simulink model "KalmanPendulumSim"  (R2018b)
settings: Solver=VariableStepAuto  StartTime=0.0  StopTime=10  FixedStep=dt  RelTol=1e-3
model workspace (MAT data in the model file):
  ControlTs = 0.01
  FNorm = 3
  L = 1
  Omega0 = 0
  OmegaNorm = 3
  Q = [0  0; 0  0.0174532925199]
  R = 1.11111111111e-07
  Theta0 = 1.0471975512
  dx = 0.001
  g = 9.81
  l = 1
  m = 1
undefined symbols (not defined in the file): DiscIntNeverNeededParam, Discrete, Time
libraries: simulink x1, sharedTrackingLibrary x1, ctrlSharedLib x1, dspsrcs4 x1, aerolibanimutils x1
settings Model: Creator=alons  LastModifiedBy=alons

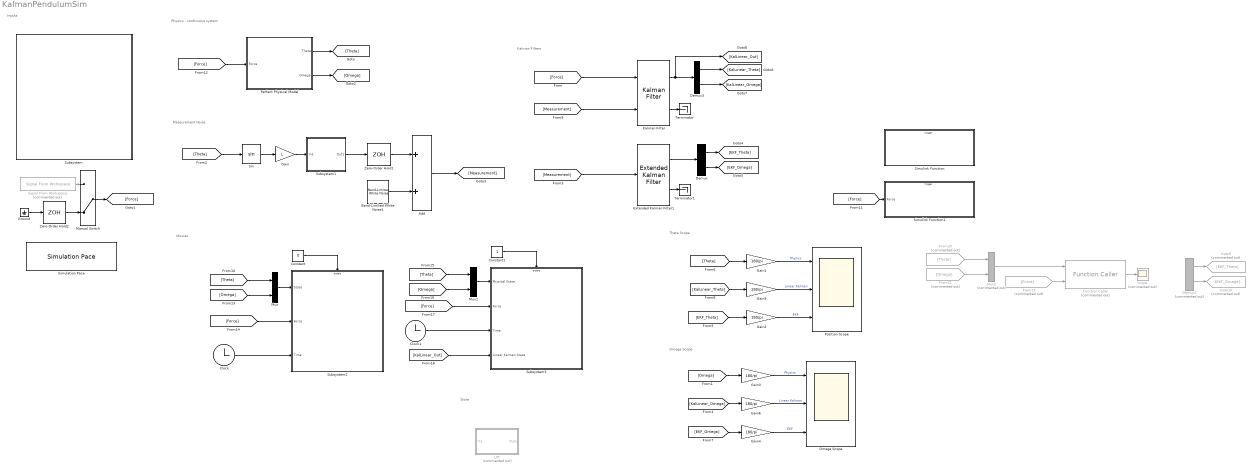
== system KalmanPendulumSim ==
  note: Store
  note: Movies
  note: Theta Scope
  note: Measurement Noise
  note: Physics - continuous system
  note: Kalman Filters
  note: Omega Scope
  note: Inputs
  Add : Sum
  Band-Limited White Noise1 : simulink/Sources/Band-Limited White Noise  Cov=R  Ts=ControlTs  seed=[23341]
  Clock : Clock
  Clock1 : Clock
  Constant : Constant  Value=0  SampleTime=0
      settings: OpenFcn=|
      | if get_param(gcbh,'value')-48
      |    set_param(gcbh,'value','0','backgroundcolor','red');
      | else
      |    set_param(gcbh,'value','1','backgroundcolor','green');
      | end
  Constant1 : Constant  SampleTime=0
      settings: OpenFcn=|
      | if get_param(gcbh,'value')-48
      |    set_param(gcbh,'value','0','backgroundcolor','red');
      | else
      |    set_param(gcbh,'value','1','backgroundcolor','green');
      | end
  Demux : Demux  Outputs=2
  Demux2 : Demux  Commented=on  Outputs=2
  Demux3 : Demux  Outputs=2
  Extended Kalman Filter1 : sharedTrackingLibrary/Extended Kalman Filter  StateTransitionFcn=StateTransition  HasStateTransitionJacobianFcn=off  HasAdditiveProcessNoise=Additive  ProcessNoise=Q  HasTimeVaryingProcessNoise=off  HasStateTransitionFcnExtraArgument=0  InitialState=[Theta0;Omega0]  InitialStateCovariance=zeros(2,2)  MeasurementFcn1=Measurement2Theta  HasMeasurementJacobianFcn1=off  HasMeasurementEnablePort1=off  HasAdditiveMeasurementNoise1=Additive  MeasurementNoise1=R  HasTimeVaryingMeasurementNoise1=off  HasMeasurementFcnExtraArgument1=0  MeasurementFcn2=myMeasurementFcn  HasMeasurementJacobianFcn2=off  HasMeasurementEnablePort2=off  HasAdditiveMeasurementNoise2=Additive  MeasurementNoise2=1  HasTimeVaryingMeasurementNoise2=off  HasMeasurementFcnExtraArgument2=0  MeasurementFcn3=myMeasurementFcn  HasMeasurementJacobianFcn3=off  HasMeasurementEnablePort3=off  HasAdditiveMeasurementNoise3=Additive  MeasurementNoise3=1  HasTimeVaryingMeasurementNoise3=off  HasMeasurementFcnExtraArgument3=0  MeasurementFcn4=myMeasurementFcn  HasMeasurementJacobianFcn4=off  HasMeasurementEnablePort4=off  HasAdditiveMeasurementNoise4=Additive  MeasurementNoise4=1  HasTimeVaryingMeasurementNoise4=off  HasMeasurementFcnExtraArgument4=0  MeasurementFcn5=myMeasurementFcn  HasMeasurementJacobianFcn5=off  HasMeasurementEnablePort5=off  HasAdditiveMeasurementNoise5=Additive  MeasurementNoise5=1  HasTimeVaryingMeasurementNoise5=off  HasMeasurementFcnExtraArgument5=0  EnableMultirate=off  StateTransitionFcnSampleTime=1  MeasurementFcn1SampleTime=1  MeasurementFcn2SampleTime=1  MeasurementFcn3SampleTime=1  MeasurementFcn4SampleTime=1  MeasurementFcn5SampleTime=1  UseCurrentEstimator=on  OutputStateCovariance=on  DataType=double  SampleTime=ControlTs  NumberOfMeasurements=1
      settings: SourceProductName=Control System Toolbox  SourceProductBaseCode=CT
  From19 : From  Commented=on  GotoTag=Force
  From20 : From  Commented=on  GotoTag=Theta
  From21 : From  Commented=on  GotoTag=Omega
  Function Caller : FunctionCaller  Commented=on  FunctionPrototype=x_kp1 = StateTransition(x_k,Force)
  Gain : Gain  Gain=L
  Gain{1..6} (6 alike) : Gain  Gain=180/pi
  Goto10 : Goto  Commented=on  GotoTag=EKF_Omega
  Goto9 : Goto  Commented=on  GotoTag=EKF_Theta
  Ground : Ground
  Kalman Filter : ctrlSharedLib/Kalman Filter  TimeDomain=Discrete-Time  UseCurrentEstimator=on  ModelSource=Individual A, B, C, D matrices  ModelSourceVariable=ss(0.95,1,1,0,1)  A=[0,1;-sqrt(g/L),0]  B=zeros(2,1)  C=[L,0]  D=0  NumberOfStates=1  NumberOfInputs=1  NumberOfOutputs=1  InitialEstimateSource=Dialog  X0=[Theta0,Omega0]  P0=10  UseK=off  UseGH=off  NumberOfProcessNoiseInputs=1  G=1  TimeInvariantG=on  H=0  TimeInvariantH=on  Q=Q  TimeInvariantQ=on  R=R  TimeInvariantR=on  N=0  TimeInvariantN=on  AddInputPort=on  AddEnablePort=off  OutputEstimatedY=off  OutputP=on  Ts=-1
      settings: SourceProductBaseCode=CT
  LPF : Subsystem  Commented=on  mask{Freq=1000}
      mask prompts: Freq "LPF Freq [Hz]"
      mask Display: fprintf('LPF %g[Hz]',Freq);
  Manual Switch : ManualSwitch  CurrentSetting=0
  Mux : Mux  Inputs=2
  Mux1 : Mux  Inputs=2
  Mux2 : Mux  Commented=on  Inputs=2
  Omega Scope : Scope  NumInputPorts=3
  Perfect Physical Model : Subsystem
  Position Scope : Scope  NumInputPorts=3
  Scope : Scope  Commented=on
  Signal From Workspace : dspsrcs4/Signal From Workspace  Commented=on  X=F  Ts=ControlTs  nsamps=1  OutputAfterFinalValue=Setting to zero  ignoreOrWarnInputAndFrameLengths=off  OutputFrames=off
  Simulation Pace : aerolibanimutils/Simulation Pace  SimulationPace=1  SleepMode=Auto  OutputPaceError=off  SampleTime=ControlTs
  Simulink Function : Subsystem  TreatAsAtomicUnit=on
  Simulink Function1 : Subsystem  TreatAsAtomicUnit=on
  Sin : Trigonometry
  Subsystem : Subsystem  InitFcn=|  mask{ControlTs=0.01, L=1, m=1, dx=1*10^-3, g=9.81, Theta0=60*pi/180, Omega0=0*pi/180, Q=diag([0,1])*pi/180, R=((1*10^-3)/3)^2, FNorm=3, OmegaNorm=3}
      | mdlWks=get_param(bdroot,'ModelWorkspace')
      | par = get_param(gcb,'DialogParameters');
      | fnames = fieldnames(par);
      | for ipar=1:length(fnames)
      |    num=str2num(get_param(gcb,fnames{ipar}));
      |    mdlWks.assignin(fnames{ipar},num);
      | end
      | 
      | clear par fnames ipar num mdlWks;
      mask prompts: ControlTs "Control Time Sample [s]"; L "String Length [m]"; m "Bolb Mass [kg]"; dx "dx - Encoder Resolution [m]"; g "g - gravity acceleration [m/s^2]"; Theta0 "Initial Theta [rad]"; Omega0 "Initial Omega [rad/s]"; Q "Q - Model Noise Covaraince [rad,rad/s]"; R "R - Measuremnt Noise Covariance"; FNorm "FNorm - for drawing [N]"; OmegaNorm "OmegaNorm - for drawing [rad/s]"
      mask Display:
      | str=[
      |     'Model Workspace Parameters \n\n\n',...
      |     'ControlTs = %g[s]\n\n',...
      |     'm = %g[kg]\n\n',...
      |     'L = %g[m]\n\n',...
      |     'dx = %g[m]\n\n\n',...
      |     'g = %g[m/s^2]\n\n',...
      |     'Theta0 = %g[rad]\n\n',...
      |     'Omega0 = %g[rad/s]\n\n',...
      |     'Q(1,1) = %g[rad]\n\n',...
      |     'Q(2,2) = %g[rad/s]\n\n',...
      |     'R = %g[m]\n\n\n',...
      |     'For Drawing\n\n',...
      |     'FNorm = %g[N]\n\n',...
      |     'OmegaNorm = %g[rad/s]',...
      |     ];
      | fprintf(str,ControlTs,m,L,dx,g,Theta0,...
      |     Omega0,Q(1,1),Q(2,2),R,FNorm,OmegaNorm);
  Subsystem1 : Subsystem
      mask Display: disp('Physics 2 Resolution')
  Subsystem2 : Subsystem
      settings: OpenFcn=|
      | UserData = get_param([gcb,'/AnimationSfcn'],'UserData');
      | Fig = UserData.Figure;
      | if ishghandle(Fig,'figure');
      |    %bring to the front:
      |    figure(Fig);
      | end
      mask Display:
      | t=linspace(0,2*pi,20);
      | plot(cos(t),sin(t));
      | 
      | x=[-0.4,-0.4,0.6,-0.4];
      | y=[-0.5,0.5,0,-0.5];
      | plot(x,y)
      | 
      | disp('Physical System')
  Subsystem3 : Subsystem
      settings: OpenFcn=|
      | UserData = get_param([gcb,'/AnimationSfcn'],'UserData');
      | Fig = UserData.Figure;
      | if ishghandle(Fig,'figure');
      |    %bring to the front:
      |    figure(Fig);
      | end
      mask Display:
      | t=linspace(0,2*pi,20);
      | plot(cos(t),sin(t));
      | 
      | x=[-0.4,-0.4,0.6,-0.4];
      | y=[-0.5,0.5,0,-0.5];
      | plot(x,y)
      | 
      | disp('Linear Kalman System')
  Terminator : Terminator
  Terminator1 : Terminator
  Zero-Order Hold1 : ZeroOrderHold  SampleTime=ControlTs
  Zero-Order Hold2 : ZeroOrderHold  SampleTime=ControlTs
  wires:
  [Theta] -> Sin/1
  Sin/1 -> Gain/1
  Extended Kalman Filter1/1 -> Demux/1
  Band-Limited White Noise1/1 -> Add/2
  Demux/1 -> [EKF_Theta]
  Demux/2 -> [EKF_Omega]
  [EKF_Theta] -> Gain2/1
  [Theta] -> Gain1/1
  Gain1/1 -> Position Scope/1  "Physics"
  [Omega] -> Gain3/1
  [EKF_Omega] -> Gain4/1
  Gain3/1 -> Omega Scope/1  "Physics"
  Demux3/1 -> [KalLinear_Theta]
  Demux3/2 -> [KalLinear_Omega]
  Kalman Filter/1 -> Demux3/1, [KalLinear_Out]
  [KalLinear_Theta] -> Gain5/1
  Gain2/1 -> Position Scope/3  "EKF"
  Gain5/1 -> Position Scope/2  "Linear Kalman"
  Gain4/1 -> Omega Scope/3  "EKF"
  [KalLinear_Omega] -> Gain6/1
  Gain6/1 -> Omega Scope/2  "Linear Kalman"
  [Measurement] -> Kalman Filter/2
  [Measurement] -> Extended Kalman Filter1/1
  Signal From Workspace/1 -> Manual Switch/1
  Ground/1 -> Zero-Order Hold2/1
  Manual Switch/1 -> [Force]
  [Force] -> Perfect Physical Model/1(Force)
  Perfect Physical Model/1(Theta) -> [Theta]
  Perfect Physical Model/2(Omega) -> [Omega]
  [Force] -> Kalman Filter/1
  Gain/1 -> Subsystem1/1(In1)
  Add/1 -> [Measurement]
  Subsystem1/1(Out1) -> Zero-Order Hold1/1
  Zero-Order Hold1/1 -> Add/1
  [Theta] -> Mux/1
  Clock/1 -> Subsystem2/3(Time)
  [Force] -> Subsystem2/2(Force)
  Mux/1 -> Subsystem2/1(State)
  [Omega] -> Mux/2
  Constant/1 -> Subsystem2/Enable
  Zero-Order Hold2/1 -> Manual Switch/2
  Constant1/1 -> Subsystem3/Enable
  [Omega] -> Mux1/2
  Clock1/1 -> Subsystem3/3(Time)
  [Theta] -> Mux1/1
  [Force] -> Subsystem3/2(Force)
  Mux1/1 -> Subsystem3/1(Physical State)
  [KalLinear_Out] -> Subsystem3/4(Linear Kalman State)
  From19/1 -> Function Caller/2
  From21/1 -> Mux2/2
  From20/1 -> Mux2/1
  Demux2/2 -> Goto10/1
  Demux2/1 -> Goto9/1
  Function Caller/1 -> Scope/1
  Mux2/1 -> Function Caller/1
  [Force] -> Simulink Function1/1(Force)
  Kalman Filter/2 -> Terminator/1
  Extended Kalman Filter1/2 -> Terminator1/1

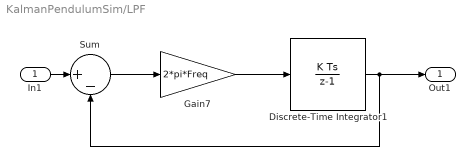
== system KalmanPendulumSim/LPF ==
  In1 : Inport
  Discrete-Time Integrator1 : DiscreteIntegrator  SampleTime=-1  ICPrevOutput=DiscIntNeverNeededParam  ICPrevScaledInput=DiscIntNeverNeededParam
  Gain7 : Gain  Gain=2*pi*Freq
  Sum : Sum  Inputs=|+-
  Out1 : Outport
  wires:
  Discrete-Time Integrator1/1 -> Out1/1, Sum/2
  Sum/1 -> Gain7/1
  Gain7/1 -> Discrete-Time Integrator1/1
  In1/1 -> Sum/1

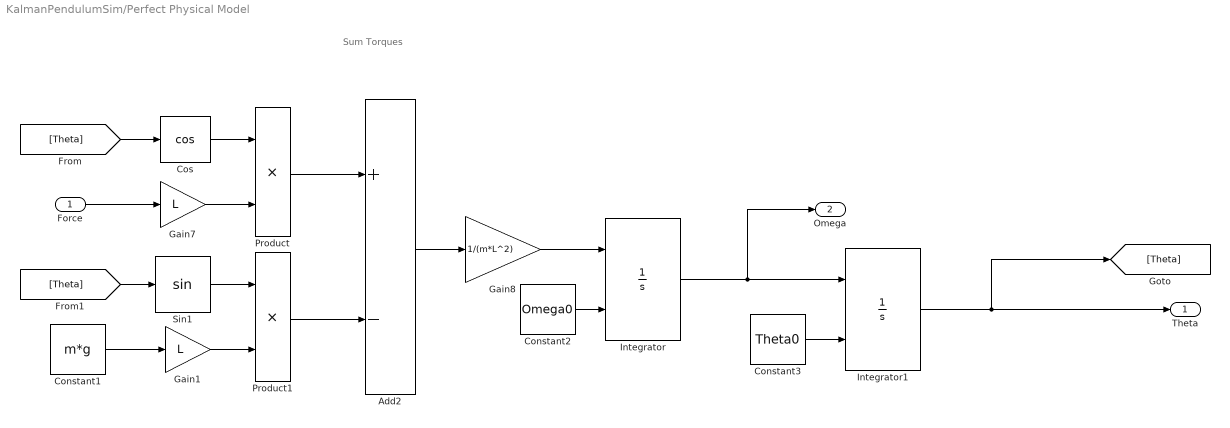
== system KalmanPendulumSim/Perfect Physical Model ==
  note: Sum Torques
  Force : Inport
  Add2 : Sum  Inputs=+-
  Constant1 : Constant  Value=m*g
  Constant2 : Constant  Value=Omega0
  Constant3 : Constant  Value=Theta0
  Cos : Trigonometry  Operator=cos
  Gain1 : Gain  Gain=L
  Gain7 : Gain  Gain=L
  Gain8 : Gain  Gain=1/(m*L^2)
  Integrator : Integrator  InitialConditionSource=external
  Integrator1 : Integrator  InitialConditionSource=external
  Product : Product
  Product1 : Product
  Sin1 : Trigonometry
  Theta : Outport
  Omega : Outport  Port=2
  wires:
  Add2/1 -> Gain8/1
  Gain8/1 -> Integrator/1
  Force/1 -> Gain7/1
  Product/1 -> Add2/1
  Gain7/1 -> Product/2
  Constant1/1 -> Gain1/1
  [Theta] -> Cos/1
  Cos/1 -> Product/1
  Product1/1 -> Add2/2
  Sin1/1 -> Product1/1
  [Theta] -> Sin1/1
  Gain1/1 -> Product1/2
  Constant2/1 -> Integrator/2
  Integrator/1 -> Omega/1, Integrator1/1
  Constant3/1 -> Integrator1/2
  Integrator1/1 -> [Theta], Theta/1

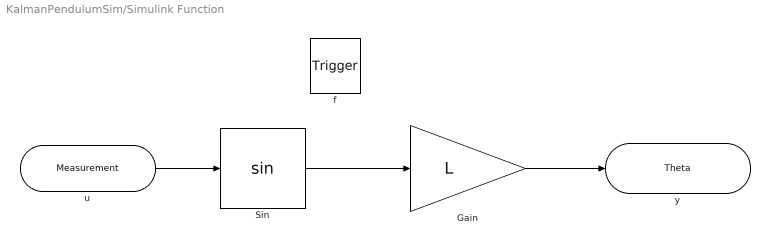
== system KalmanPendulumSim/Simulink Function ==
  f : TriggerPort  TriggerType=function-call  IsSimulinkFunction=on  FunctionName=Measurement2Theta  FunctionVisibility=scoped  VariantControl=(inherit)
  Gain : Gain  Gain=L
  Sin : Trigonometry
  u : ArgIn  DisableCoverage=on  ArgumentName=Measurement
  y : ArgOut  DisableCoverage=on  ArgumentName=Theta
  wires:
  u/1 -> Sin/1
  Sin/1 -> Gain/1
  Gain/1 -> y/1

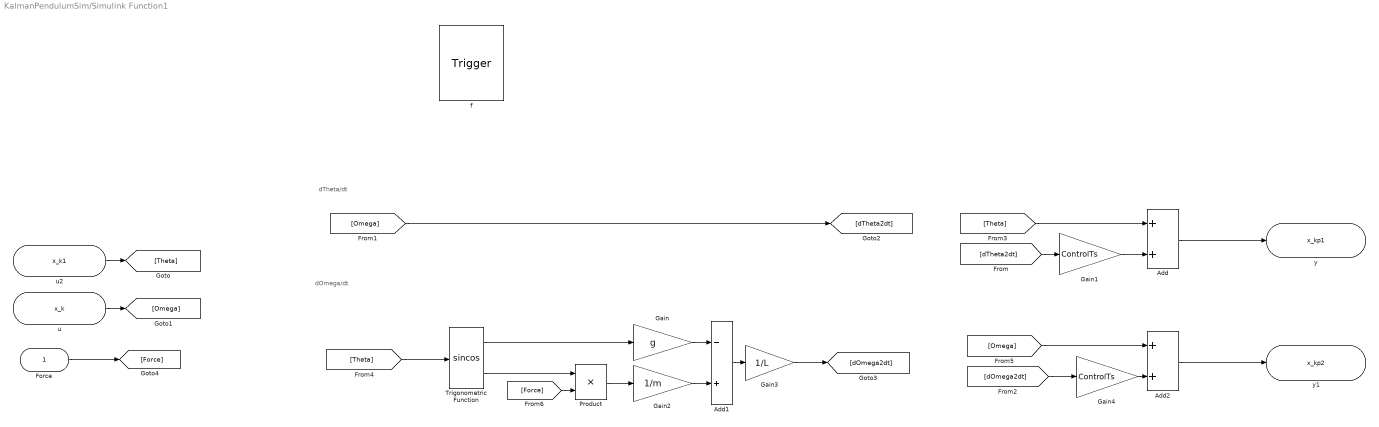
== system KalmanPendulumSim/Simulink Function1 ==
  note: dTheta/dt
  note: dOmega/dt
  Force : Inport
  f : TriggerPort  TriggerType=function-call  IsSimulinkFunction=on  FunctionName=StateTransition  FunctionVisibility=scoped  VariantControl=(inherit)
  Add : Sum
  Add1 : Sum  Inputs=-+
  Add2 : Sum
  Gain : Gain  Gain=g
  Gain1 : Gain  Gain=ControlTs
  Gain2 : Gain  Gain=1/m
  Gain3 : Gain  Gain=1/L
  Gain4 : Gain  Gain=ControlTs
  Product : Product
  Trigonometric Function : Trigonometry  Operator=sincos
  u : ArgIn  DisableCoverage=on  ArgumentName=x_k
  u2 : ArgIn  DisableCoverage=on  Port=2  ArgumentName=x_k1
  y : ArgOut  DisableCoverage=on  ArgumentName=x_kp1
  y1 : ArgOut  DisableCoverage=on  Port=2  ArgumentName=x_kp2
  wires:
  u2/1 -> [Theta]
  u/1 -> [Omega]
  [Omega] -> [dTheta2dt]
  Add/1 -> y/1
  [dTheta2dt] -> Gain1/1
  Gain1/1 -> Add/2
  [Theta] -> Add/1
  Gain2/1 -> Add1/2
  Trigonometric Function/1 -> Gain/1
  Add1/1 -> Gain3/1
  Gain/1 -> Add1/1
  [Theta] -> Trigonometric Function/1
  Trigonometric Function/2 -> Product/1
  Product/1 -> Gain2/1
  Gain3/1 -> [dOmega2dt]
  [Force] -> Product/2
  [dOmega2dt] -> Gain4/1
  Gain4/1 -> Add2/2
  [Omega] -> Add2/1
  Add2/1 -> y1/1
  Force/1 -> [Force]

== system KalmanPendulumSim/Subsystem ==

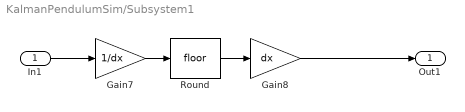
== system KalmanPendulumSim/Subsystem1 ==
  In1 : Inport
  Gain7 : Gain  Gain=1/dx
  Gain8 : Gain  Gain=dx
  Round : Rounding
  Out1 : Outport
  wires:
  Gain7/1 -> Round/1
  Gain8/1 -> Out1/1
  Round/1 -> Gain8/1
  In1/1 -> Gain7/1

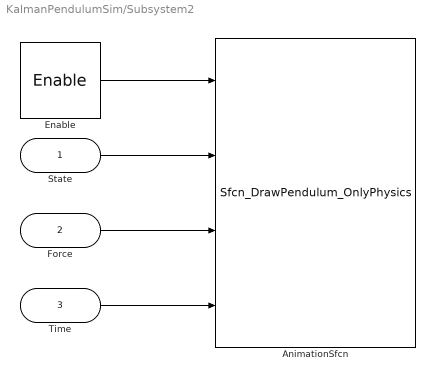
== system KalmanPendulumSim/Subsystem2 ==
  State : Inport
  Force : Inport  Port=2
  Time : Inport  Port=3
  Enable : EnablePort  StatesWhenEnabling=reset  ShowOutputPort=on
  AnimationSfcn : M-S-Function  FunctionName=Sfcn_DrawPendulum_OnlyPhysics  Parameters=ControlTs,[-2*L,2*L],[-2*L,L/2],L,g,m,FNorm,OmegaNorm
  wires:
  Time/1 -> AnimationSfcn/4
  Force/1 -> AnimationSfcn/3
  State/1 -> AnimationSfcn/2
  Enable/1 -> AnimationSfcn/1

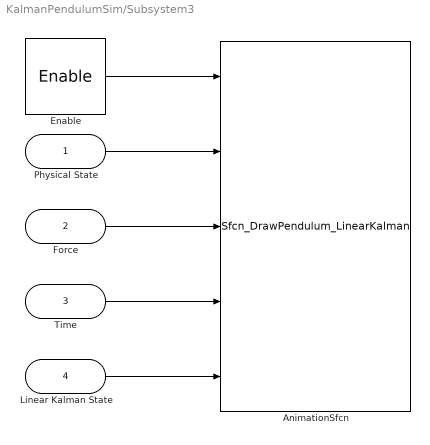
== system KalmanPendulumSim/Subsystem3 ==
  Physical State : Inport
  Force : Inport  Port=2
  Time : Inport  Port=3
  Linear Kalman State : Inport  Port=4
  Enable : EnablePort  StatesWhenEnabling=reset  ShowOutputPort=on
  AnimationSfcn : M-S-Function  FunctionName=Sfcn_DrawPendulum_LinearKalman  Parameters=ControlTs,[-2*L,2*L],[-2*L,L/2],L,g,m,FNorm,OmegaNorm
  wires:
  Time/1 -> AnimationSfcn/4
  Force/1 -> AnimationSfcn/3
  Physical State/1 -> AnimationSfcn/2
  Enable/1 -> AnimationSfcn/1
  Linear Kalman State/1 -> AnimationSfcn/5
